simulink model "simpleMicrogrid_PhasorEMT"  (R2017b)
settings: Solver=ode23tb  StartTime=0.0  StopTime=60  RelTol=1e-3
InitFcn:
  | Ts = 1e-4;
  | Rs = 4;
  | Ls = 0;
  | kv = 1;
undefined symbols (not defined in the file): DiscIntNeverNeededParam, Tlim
libraries: powerlib x65, powerlib_meascontrol x7, simulink x6, sps_avr x1, spsDieselMotorModel x1
(part 1 of 2)
settings Model: SimulationMode=accelerator  Creator=jlesage  LastModifiedBy=jlesage
settings DebuggingCC: UnconnectedInputMsg=none  UnconnectedOutputMsg=none  UnconnectedLineMsg=none

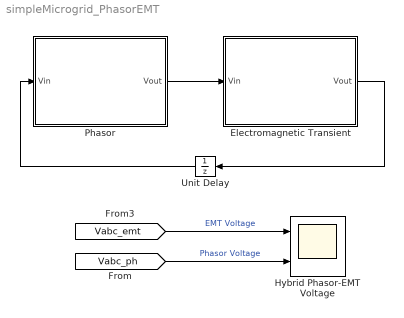
== system simpleMicrogrid_PhasorEMT ==
  Electromagnetic Transient : Subsystem
  Hybrid Phasor-EMT Voltage : Scope  NumInputPorts=2
  Phasor : Subsystem
  Unit Delay : UnitDelay  SampleTime=Ts
  wires:
  Phasor/1(Vout) -> Electromagnetic Transient/1(Vin)
  Electromagnetic Transient/1(Vout) -> Unit Delay/1
  Unit Delay/1 -> Phasor/1(Vin)
  [Vabc_emt] -> Hybrid Phasor-EMT Voltage/1  "EMT Voltage"
  [Vabc_ph] -> Hybrid Phasor-EMT Voltage/2  "Phasor Voltage"

== system simpleMicrogrid_PhasorEMT/Electromagnetic Transient ==
  Vin : Inport  SampleTime=Ts
  Energy Storage : Subsystem  mask(Grid-connected Energy Storage (PQ Model)){Vn=5000, Fn=60, PnomkW=500, kWh_Rated=100, Efficiency=96, LimitVec=[90 10], RechargeSOC=11, Precharge=50, autoRecharge=off, Initial_kWh_pc=80, PQvec=[500e3 0]}
      mask prompts: Vn "Nominal L-L Voltage [Vrms]"; Fn "Nominal Frequency [Hz]"; PnomkW "Rated Power [kW]"; kWh_Rated "Rated Capacity [kWh]"; Efficiency "Overall System Efficiency [%]"; LimitVec "Upper/Lower Charge Limits [%]"; RechargeSOC "SOC to Recharge [%]"; Precharge "Recharge Rate [% of Rated Power]"; autoRecharge "Enable Auto-Recharge"; Initial_kWh_pc "Initial State-of-Charge [0-100%]"; PQvec "Initial Active/Reactive Cmds"
      mask help:
      | The energy storage block models a generic grid-connected energy storage system (ESS), most commonly a battery system. This is a system-level model that does not contain any power electronics, but is useful for load flow, phasor, and hybrid phasor-EMT simulations. The inputs to this block are the commanded active and reactive power of the ESS. The ESS is assumed to have four quadrent operation.
      |
      | For more detailed ESS models, consider the battery block in the Drives library. Consider using this PQ Model to perform load flow studies and switch to a more detailed model when full EMT studies or more advanced controls are required.
      |
      | Note: The initial active/reactive power commands must be specified for use for Load Flow analysis.
      mask init:
      | % Calculate Initial Conditions
      | Pnom = PnomkW*1e3;
      | P0 = -PQvec(1);  Q0 = -PQvec(2);
      | if abs(P0) > Pnom
      |     P0 = sign(P0)*Pnom;
      | end
      | 
      | % Calculate Q0 given Reactive Power Capability Curve
      | Qlim = sqrt(Pnom^2 - P0^2);
      | if Qlim > abs(Q0)
      |     Q0 = sign(Q0)*Qlim;
      | end
      | 
      | UpChrgLim = LimitVec(1);
      | LowChrgLim = LimitVec(2);
      | if Initial_kWh_pc > UpChrgLim && P0 < 0
      |     P0 = 0; Q0 = 0;
      | elseif Initial_kWh_pc < LowChrgLim && P0 > 0
      |     P0 = 0; Q0 = 0;
      | end
      mask DialogControl Container7 Prompt: Grid Connection Properties
      mask DialogControl Container11 Prompt: Charge/Discharge Controls
      mask DialogControl Container12 Prompt: Initial Conditions
  Pref : Constant  Value=100e3
  Qref : Constant  Value=0
  SPS-Simulink Interface : Subsystem  Variant=on  OverrideUsingVariant=EMT  mask(SPS-to-Simulink Voltage Interface){replayType=EMT Replay, Freq=60, kv=kv, Rs=Rs, Ls=Ls, Ts=Ts}
      mask prompts: replayType "Replay Type"; Freq "Nominal Frequency [Hz]"; kv "Voltage Stability Factor, kv"; Rs "Series Resistance, Rs"; Ls "Series Inductance, Ls"; Ts "Sample Time, Ts"
      mask help:
      | This block uses voltage transfer theory to segment a Simscape Power Systems network into subsystems. These subsystems can execute a multiple rates, use Phasor/EMT simulation methods, and run on multiple cores for real-time simulation.
      |
      | Make sure to select the same simulation technique as the powergui setting in the same subsystem.
      mask init:
      | simulationStatus =  get_param(bdroot,'SimulationStatus');
      | 
      | % The active variant can only be modified at edit-time or very early during
      | % the simulink compile stage. 
      | if any(strcmp(simulationStatus, {'stopped'}))
      |     vssBlk = gcb;
      |     freqBlk = [vssBlk '/EMT/Frequency Generator'];
      | 
      |     if strcmp(replayType,'EMT Replay')
      |         set_param(vssBlk, 'OverrideUsingVariant', 'EMT');
      |     else
      |         set_param(vssBlk, 'OverrideUsingVariant', 'Phasor');
      |     end
      |     
      |     if Ts ~= 0
      |         set_param(freqBlk,'OverrideUsingVariant', 'Discrete');
      |     else
      |         set_param(freqBlk, 'OverrideUsingVariant', 'Continuous');
      |     end
      | end
      mask TypeOptions replayType: EMT Replay | Phasor Replay
  Scope : Subsystem
  Three-Phase V-I Measurement : powerlib/Measurements/Three-Phase V-I Measurement  VoltageMeasurement=phase-to-ground  SetLabelV=on  LabelV=Vabc_ess  Vpu=off  VpuLL=off  CurrentMeasurement=yes  SetLabelI=on  LabelI=Iabc_ess  Ipu=off  Pbase=100e6  Vbase=500e3  OutputType=Complex  PhasorSimulation=on  PSBequivalent=0
  powergui : powerlib/powergui  Priority=1  SimulationMode=Discrete  SampleTime=Ts  frequency=60  Iterations=50  frequencyindice=60  Pbase=100e6  ErrMax=0.0001  UnitsV=kV  UnitsW=MW  buscounter=3  FunctionMessages=off  echomessages=off  EnableUseOfTLC=off  CurrentSourceSwitches=off  DisableSnubberDevices=off  DisableRonSwitches=off  DisableVfSwitches=off  DisplayEquations=off  SolverType=Tustin/Backward Euler (TBE)  Interpol=off  ExternalGateDelay=off  methode=off  Ts=100  x0status=blocks  SPID=on  SwTol=0  HookPort=off  RestoreLinks=warning  ResistiveCurrentMeasurement=off  Frange=[0:2:500]  Ylog=off  Xlog=on  ShowGrid=off  save=off  variable=ZData  structure=0  ZoomFFT=off  StartTime=0.0  cycles=1  DisplayStyle=1  fundamental=60  FreqAxis=off  MaxFrequency=1000  frequencyindicesteady=1  RmsSteady=1  display=off
  Vout : Outport  SampleTime=Ts
  tag scope: battM=global
  wires:
  SPS-Simulink Interface/1(Vout) -> Vout/1
  Vin/1 -> SPS-Simulink Interface/1(Vin)
  [Vabc_ess] -> Scope/1(Vrms)
  Energy Storage/1(m) -> [battM]
  Pref/1 -> Energy Storage/1(Pref)
  Qref/1 -> Energy Storage/2(Qref)
  connections:
  Three-Phase V-I Measurement/RConn1 -- Energy Storage/RConn1
  Three-Phase V-I Measurement/RConn2 -- Energy Storage/RConn2
  Three-Phase V-I Measurement/RConn3 -- Energy Storage/RConn3
  Three-Phase V-I Measurement/LConn3 -- SPS-Simulink Interface/RConn3
  Three-Phase V-I Measurement/LConn2 -- SPS-Simulink Interface/RConn2
  Three-Phase V-I Measurement/LConn1 -- SPS-Simulink Interface/RConn1

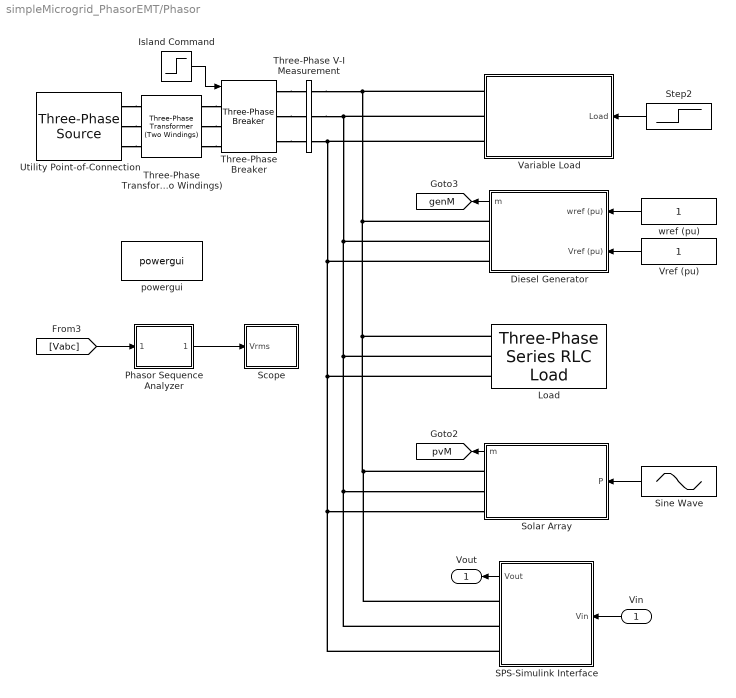
== system simpleMicrogrid_PhasorEMT/Phasor ==
  Vin : Inport
  Diesel Generator : Subsystem  mask(Diesel Generator (Simple)){Pn=1e6, Vn=5000, Fn=60, genType=PQ, PQ0=[0.05 0]}
      mask prompts: Pn "Generator Rated Power [W]"; Vn "Rated Voltage [V]"; Fn "Rated Frequency [Hz]"; genType "Load Flow Type"; PQ0 "Initial Power, [P0 Q0] [pu]"
      mask help:
      | The Diesel Generator block contains a synchronous generator, diesel governor and excitation system to represent the dynamics of a Genset. To inspect the model, look under the block mask (Ctrl + u).
      |
      | The inputs to the basic Diesel generator block are the desired speed reference (in pu) and the desired voltage reference (in pu). The output measurements are contained in a Simulink bus, which can be selected by using the Bus Selector block.
      |
      | Note: The initial generator power must be specified for use for Load Flow analysis.
      mask init:
      | % Extract Initial Active/Reactive Power
      | P0 = PQ0(1);
      | Q0 = PQ0(2);
      | 
      | % Select Load Flow Type
      | genBlock = [gcb '/Synchronous Machine'];
      | currentVals = get_param(genBlock,'MaskValues');
      | currentVals{31} = genType;
      | set_param(genBlock,'MaskValues',currentVals);
      | 
      | % Disable Option if Swing Generator Selected
      | currentEnables = get_param(gcb,'MaskEnables');
      | if strcmp(genType,'swing')
      |     currentEnables{5} = 'off';
      | else
      |     currentEnables{5} = 'on';
      | end
      | set_param(gcb,'MaskEnables',currentEnables);
      settings: AttributesFormatString=Rated Power: %<Pn> W
      mask TypeOptions genType: swing | PQ | PV
      mask Display: %image(imread('diesel.jpg'))
  Island Command : Step  Time=15  Before=1  After=0  SampleTime=0
  Load : powerlib/Elements/Three-Phase Series RLC Load  LConnTagsString=A|B|C  Configuration=Y (grounded)  NominalVoltage=5000  Vabc=[1e3 1e3 1e3]  Vabcp=[1e3 1e3 1e3]  NominalFrequency=60  UnbalancedPower=off  ActivePower=500e3  InductivePower=0  CapacitivePower=0  Pabc=[10e3 9e3 11e3]  QLabc=[100 90 110]  QCabc=[100 90 110]  Pabcp=[10e3 9e3 11e3]  QLabcp=[100 90 110]  QCabcp=[100 90 110]  Measurements=None  LoadType=constant Z
      settings: AttributesFormatString=P = %<ActivePower> W
  Phasor Sequence Analyzer : Subsystem
  SPS-Simulink Interface : Subsystem  Variant=on  OverrideUsingVariant=Phasor  mask(SPS-to-Simulink Voltage Interface){replayType=Phasor Replay, Freq=60, kv=kv, Rs=Rs, Ls=Ls, Ts=Ts}
      mask prompts: replayType "Replay Type"; Freq "Nominal Frequency [Hz]"; kv "Voltage Stability Factor, kv"; Rs "Series Resistance, Rs"; Ls "Series Inductance, Ls"; Ts "Sample Time, Ts"
      mask help:
      | This block uses voltage transfer theory to segment a Simscape Power Systems network into subsystems. These subsystems can execute a multiple rates, use Phasor/EMT simulation methods, and run on multiple cores for real-time simulation.
      |
      | Make sure to select the same simulation technique as the powergui setting in the same subsystem.
      mask init: same as simpleMicrogrid_PhasorEMT/Electromagnetic Transient/SPS-Simulink Interface
      mask TypeOptions replayType: EMT Replay | Phasor Replay
  Scope : Subsystem
  Sine Wave : Sin  Amplitude=200e3  Bias=250e3  Frequency=0.05  SampleTime=0
  Solar Array : Subsystem  mask(Grid-Connected PV Array (PQ Model)){Vn=5000, Fn=60, P0=500e3}
      mask prompts: Vn "Nominal L-L Voltage [Vrms]"; Fn "Nominal Frequency [Hz]"; P0 "Initial Power [W]"
      mask help:
      | This block models a grid-connected solar array using the Three-Phase Dynamic Load block. This is a system-level model that does not contain any power electronics, but is useful for load flow, phasor, and hybrid phasor-EMT simulations. The input to this block is the power output of the grid connected PV array, not irradiance.
      |
      | For more detailed PV models, consider the PV Array block in the Renewables library. Consider using this PQ Model to perform load flow studies and switch to a more detailed model when full EMT studies are required.
      |
      | Note: The array power must be specified for use for Load Flow analysis.
      mask init:
      | % P0 = Irr0*TotalArea*Efficiency/100;
      | P0 = -P0;
      mask Display:
      | image(imread('PV_Farm.jpg'))
      | color('white')
      | port_label('input',1,'P')
      | port_label('output',1,'m')
      | port_label('Rconn',1,'A')
      | port_label('Rconn',2,'B')
      | port_label('Rconn',3,'C')
  Step2 : Step  Time=35  Before=200e3  After=500e3  SampleTime=0
  Three-Phase Transformer (Two Windings) : powerlib/Elements/Three-Phase Transformer (Two Windings)  Winding1Connection=Yg  Winding2Connection=Yg  CoreType=Three single-phase transformers  SetSaturation=off  Hysteresis=off  DataFile='hysteresis'  SetInitialFlux=off  Measurements=None  UNITS=pu  NominalPower=[ 250e6 , 60 ]  Winding1=[ 13.8e3 , 0.002 , 0.08 ]  Winding2=[ 5000 , 0.002 , 0.08 ]  Rm=500  Lm=500  L0=0.5  Saturation=[ 0,0 ; 0.0024,1.2 ; 1.0,1.52 ]  InitialFluxes=[ 0.8 , -0.8 , 0.7 ]  MoreParameters=off  BreakLoop=off  DataType=off  TransfoNumber=1
  Three-Phase V-I Measurement : powerlib/Measurements/Three-Phase V-I Measurement  VoltageMeasurement=phase-to-ground  SetLabelV=on  LabelV=Vabc  Vpu=off  VpuLL=off  CurrentMeasurement=yes  SetLabelI=on  LabelI=Iabc  Ipu=off  Pbase=100e6  Vbase=500e3  OutputType=Complex  PhasorSimulation=on  PSBequivalent=0
  Three-Phase Breaker : powerlib/Elements/Three-Phase Breaker  InitialState=closed  SwitchA=on  SwitchB=on  SwitchC=on  SwitchTimes="[1/60  5/60]"  External=on  BreakerResistance=0.01  SnubberResistance=1e6  SnubberCapacitance=inf  Measurements=None
  Utility Point-of-Connection : powerlib/Electrical Sources/Three-Phase Source  InternalConnection=Yg  VoltagePhases=off  Voltage=(13800)*1.00243  PhaseAngle=0.071468  Voltage_phases=[25e3 25e3 25e3]/sqrt(3)  PhaseAngles_phases=[0 -120 +120]  Frequency=60  NonIdealSource=on  SpecifyImpedance=on  Resistance=0.8929  Inductance=16.58e-3  ShortCircuitLevel=250e6  BaseVoltage=13.8e3  XRratio=7  BusType=swing  Pref=10e3  Qref=0  Prefabc=[10e3, 10e3, 10e3]  Qrefabc=[0, 0, 0]  Qmin=-inf  Qmax=inf
  Variable Load : Subsystem  mask(Variable Load (PQ Model)){Vn=5000, Fn=60, PF=1, Load0=200e3}
      mask prompts: Vn "Nominal L-L Voltage [Vrms]"; Fn "Nominal Frequency [Hz]"; PF "Power Factor [0 to 1]"; Load0 "Initial Load [W]"
      mask help:
      | The Variable Load block is a lumped approximation for a distribution feeder. For non-unity power factor loads, the input (active power) is scaled accordingly to generate a desired load.
      |
      | Note: The initial input load must be specified for use for Load Flow analysis.
      mask init:
      | P0 = Load0;
      | Q0 = Load0*sqrt(1/PF-1);
      mask Display:
      | image(imread('Residential.jpg'))
      | color('white')
      | port_label('input',1,'Load')
      | port_label('Rconn',1,'A')
      | port_label('Rconn',2,'B')
      | port_label('Rconn',3,'C')
  Vref (pu) : Constant
  powergui : powerlib/powergui  Priority=1  SimulationMode=Phasor  SampleTime=1e-4  frequency=60  Iterations=50  frequencyindice=60  Pbase=100e6  ErrMax=0.0001  UnitsV=kV  UnitsW=MW  buscounter=3  FunctionMessages=off  echomessages=off  EnableUseOfTLC=off  CurrentSourceSwitches=off  DisableSnubberDevices=off  DisableRonSwitches=off  DisableVfSwitches=off  DisplayEquations=off  SolverType=Tustin/Backward Euler (TBE)  Interpol=off  ExternalGateDelay=off  methode=off  Ts=100  x0status=blocks  SPID=on  SwTol=0  HookPort=off  RestoreLinks=warning  ResistiveCurrentMeasurement=off  Frange=[0:2:500]  Ylog=off  Xlog=on  ShowGrid=off  save=off  variable=ZData  structure=0  ZoomFFT=off  StartTime=0.0  cycles=1  DisplayStyle=1  fundamental=60  FreqAxis=off  MaxFrequency=1000  frequencyindicesteady=1  RmsSteady=1  display=off
  wref (pu) : Constant
  Vout : Outport
  tag scope: genM=global, pvM=global
  wires:
  Vref (pu)/1 -> Diesel Generator/2(Vref (pu))
  wref (pu)/1 -> Diesel Generator/1(wref (pu))
  Island Command/1 -> Three-Phase Breaker/1
  Sine Wave/1 -> Solar Array/1(P)
  Phasor Sequence Analyzer/1(Vrms) -> Scope/1(Vrms)
  [Vabc] -> Phasor Sequence Analyzer/1(Vabc)
  Diesel Generator/1(m) -> [genM]
  Step2/1 -> Variable Load/1(Load)
  Solar Array/1(m) -> [pvM]
  Vin/1 -> SPS-Simulink Interface/1(Vin)
  SPS-Simulink Interface/1(Vout) -> Vout/1
  connections:
  Utility Point-of-Connection/RConn1 -- Three-Phase Transformer (Two Windings)/LConn1
  Utility Point-of-Connection/RConn3 -- Three-Phase Transformer (Two Windings)/LConn3
  Three-Phase Transformer (Two Windings)/RConn1 -- Three-Phase Breaker/LConn1
  Three-Phase Transformer (Two Windings)/RConn2 -- Three-Phase Breaker/LConn2
  Utility Point-of-Connection/RConn2 -- Three-Phase Transformer (Two Windings)/LConn2
  Three-Phase Transformer (Two Windings)/RConn3 -- Three-Phase Breaker/LConn3
  Variable Load/RConn1 -- Three-Phase V-I Measurement/RConn1 -- Load/LConn1 -- SPS-Simulink Interface/RConn1 -- Solar Array/RConn1 -- Diesel Generator/RConn1
  SPS-Simulink Interface/RConn2 -- Solar Array/RConn2 -- Load/LConn2 -- Three-Phase V-I Measurement/RConn2 -- Variable Load/RConn2 -- Diesel Generator/RConn2
  SPS-Simulink Interface/RConn3 -- Solar Array/RConn3 -- Load/LConn3 -- Three-Phase V-I Measurement/RConn3 -- Variable Load/RConn3 -- Diesel Generator/RConn3
  Three-Phase Breaker/RConn1 -- Three-Phase V-I Measurement/LConn1
  Three-Phase Breaker/RConn3 -- Three-Phase V-I Measurement/LConn3
  Three-Phase Breaker/RConn2 -- Three-Phase V-I Measurement/LConn2

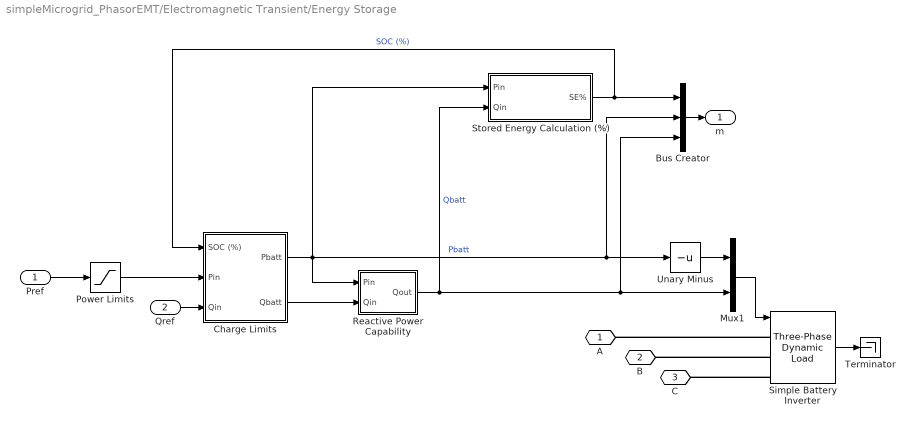
== system simpleMicrogrid_PhasorEMT/Electromagnetic Transient/Energy Storage ==
  Pref : Inport  SampleTime=Ts
  Qref : Inport  Port=2  SampleTime=Ts
  Bus Creator : BusCreator  Inputs=3
  Charge Limits : Subsystem
  Mux1 : Mux  Inputs=2
  Power Limits : Saturate  UpperLimit=Pnom  LowerLimit=-Pnom
  Reactive Power Capability : Subsystem
  Simple Battery Inverter : powerlib/Elements/Three-Phase Dynamic Load  NominalVoltage=[Vn Fn]  ActiveReactivePowers=[-500000 -3.38813e-13]  PositiveSequence=[0.999844 -0.0038635]  ExternalControl=on  NpNq=[1.3 2]  TimeConstants="[0  0  0  0]"  MinimumVoltage=0.7  Tfilter=1e-2  LoadFlowParameters=[4,0,0,0,0]
      settings: SourceProductName=Simscape Power Systems  SourceProductBaseCode=PS
  Stored Energy Calculation (%) : Subsystem
  Terminator : Terminator
  Unary Minus : UnaryMinus
  A : PMIOPort  Port=1  Side=Right
  B : PMIOPort  Port=2  Side=Right
  C : PMIOPort  Port=3  Side=Right
  m : Outport
  wires:
  Charge Limits/2(Qbatt) -> Reactive Power Capability/2(Qin)
  Qref/1 -> Charge Limits/3(Qin)
  Power Limits/1 -> Charge Limits/2(Pin)
  Charge Limits/1(Pbatt) -> Reactive Power Capability/1(Pin), Unary Minus/1, Bus Creator/2, Stored Energy Calculation (%)/1(Pin)  "Pbatt"
  Stored Energy Calculation (%)/1(SE%) -> Bus Creator/1, Charge Limits/1(SOC (%))  "SOC (%)"
  Bus Creator/1 -> m/1
  Pref/1 -> Power Limits/1
  Reactive Power Capability/1(Qout) -> Mux1/2, Bus Creator/3, Stored Energy Calculation (%)/2(Qin)  "Qbatt"
  Simple Battery Inverter/1 -> Terminator/1
  Mux1/1 -> Simple Battery Inverter/1
  Unary Minus/1 -> Mux1/1
  connections:
  Simple Battery Inverter/LConn1 -- A/RConn1
  Simple Battery Inverter/LConn3 -- C/RConn1
  Simple Battery Inverter/LConn2 -- B/RConn1

== system simpleMicrogrid_PhasorEMT/Electromagnetic Transient/SPS-Simulink Interface ==
  Vin : Inport
  EMT : Subsystem  VariantControl=EMT
  Phasor : Subsystem  VariantControl=Phasor
  A : PMIOPort  Port=1  Side=Right
  B : PMIOPort  Port=2  Side=Right
  C : PMIOPort  Port=3  Side=Right
  Vout : Outport

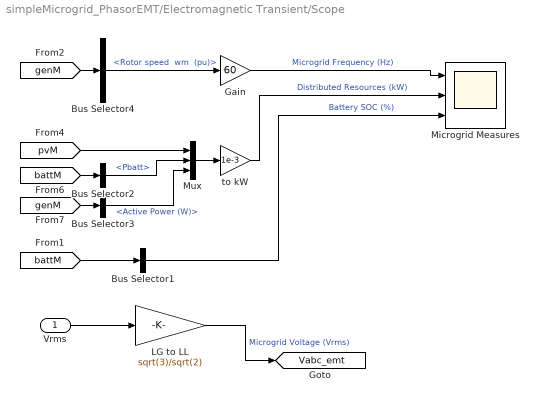
== system simpleMicrogrid_PhasorEMT/Electromagnetic Transient/Scope ==
  Vrms : Inport
  Bus Selector1 : BusSelector  OutputSignals=SOC (%)  OutputAsBus=on
  Bus Selector2 : BusSelector  OutputSignals=Pbatt
  Bus Selector3 : BusSelector  OutputSignals=Active Power (W)
  Bus Selector4 : BusSelector  OutputSignals="Rotor speed  wm  (pu)"
  Gain : Gain  Gain=60
  LG to LL : Gain  Gain=sqrt(3)/sqrt(2)
  Microgrid Measures : Scope  NumInputPorts=3
  Mux : Mux  Inputs=3
  to kW : Gain  Gain=1e-3
  tag scope: Vabc_emt=global
  wires:
  Vrms/1 -> LG to LL/1
  LG to LL/1 -> [Vabc_emt]  "Microgrid Voltage (Vrms)"
  Mux/1 -> to kW/1
  [pvM] -> Mux/1
  Bus Selector2/1 -> Mux/2  "<Pbatt>"
  [battM] -> Bus Selector2/1
  [genM] -> Bus Selector3/1
  [battM] -> Bus Selector1/1
  Bus Selector1/1 -> Microgrid Measures/3  "Battery SOC (%)"
  Gain/1 -> Microgrid Measures/1  "Microgrid Frequency (Hz)"
  [genM] -> Bus Selector4/1
  Bus Selector4/1 -> Gain/1  "<Rotor speed  wm  (pu)>"
  to kW/1 -> Microgrid Measures/2  "Distributed Resources (kW)"
  Bus Selector3/1 -> Mux/3  "<Active Power (W)>"

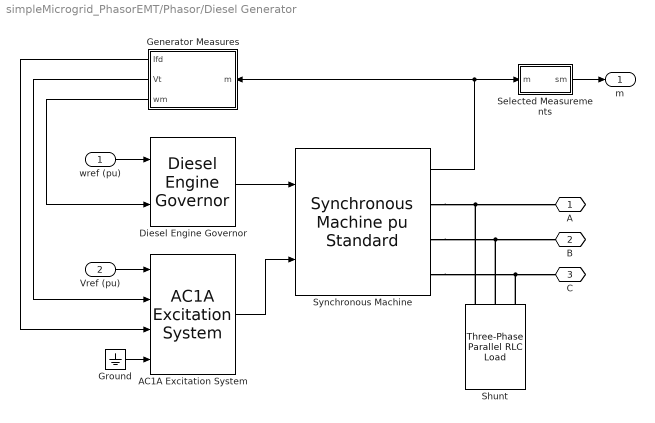
== system simpleMicrogrid_PhasorEMT/Phasor/Diesel Generator ==
  wref (pu) : Inport
  Vref (pu) : Inport  Port=2
  AC1A Excitation System : sps_avr/AC1A Excitation System  Tr=20e-3  KaTa=[400 0.02]  VAminmax=[-14.5 14.5]  VRminmax=[-5.43 6.03]  KfTf=[0.03 1.0]  TbTc=[0 0]  KeTe=[1.0 0.80]  Ve12=[4.18 3.14]  SeVe12=[0.10 0.03]  Kd=0.38  Kc=0.20  v0=[0.99984 1.0013]  TsBlock=0
      settings: SourceProductName=Simscape Power Systems  SourceProductBaseCode=PS
  Diesel Engine Governor : spsDieselMotorModel/Diesel Engine Governor  K=29  Tr=[0.01 0.02 0.2]  Ta=[0.25 0.009 0.0384]  Tlim=[0 1.1]  Td=0.024  Pm0=0.050008
  Generator Measures : Subsystem
  Ground : Ground
  Selected Measurements : Subsystem
  Shunt : powerlib/Elements/Three-Phase Parallel RLC Load  LConnTagsString=A|B|C  Configuration=Y (grounded)  NominalVoltage=Vn  Vabc=[1e3 1e3 1e3]  Vabcp=[1e3 1e3 1e3]  NominalFrequency=Fn  UnbalancedPower=off  ActivePower=Pn*0.05  InductivePower=0  CapacitivePower=0  Pabc=[10e3 9e3 11e3]  QLabc=[100 90 110]  QCabc=[100 90 110]  Pabcp=[10e3 9e3 11e3]  QLabcp=[100 90 110]  QCabcp=[100 90 110]  Measurements=None  LoadType=constant Z
  Synchronous Machine : powerlib/Machines/Synchronous Machine pu Standard  PresetModel=No  MechanicalLoad=Mechanical power Pm  ShowDetailedParameters=on  RotorType=Salient-pole  Units=per unit standard parameters  MeasurementBus=off  NominalParameters=[ Pn Vn Fn]  Reactances1=[ 1.81, 0.3, 0.23, 1.76, 0.65, 0.25, 0.15 ]  Reactances2="[ 1.305, 0.296, 0.252, 0.474,  0.243,  0.18 ]"  dAxisTimeConstants=Open-circuit  qAxisTimeConstants=Short-circuit  TimeConstants1="[ 4.4849  0.0681  0.1  ]"  TimeConstants2=[ 8.0, 0.03, 1.0, 0.07 ]  TimeConstants3="[  4.49  0.0681  0.0513  ]"  TimeConstants4=[ 8.0, 0.03, 0.3371, 0.0295 ]  TimeConstants5=[ 1.01, 0.053, 0.1 ]  TimeConstants6=[ 1.3201, 0.023, 1.0, 0.07 ]  TimeConstants7=[0.012 0.003 0.003]  TimeConstants8=[ 1.3201, 0.0231, 0.3371, 0.0295 ]  StatorResistance=0.003  Mechanical=[3.7 0 1 ]  PolePairs=20  InitialConditions=[0 -88.646 0.0500078 0.0500078 0.0500078 -0.0038635 -120.004 119.996 1.00126]  SetSaturation=off  Saturation=[0.6404,0.7127,0.8441,0.9214,0.9956,1.082,1.19,1.316,1.457;0.7,0.7698,0.8872,0.9466,0.9969,1.046,1.1,1.151,1.201]  LoadFlowParameters=[1,0,0,0,0]  TsPowergui=0  TsBlock=-1  IterativeModel=Trapezoidal non iterative  IterativeDiscreteModel=Trapezoidal non iterative  BusType=PQ  Pref=Pn*P0  Qref=0  Qmin=-inf  Qmax=inf  PLF=0  QLF=0
      settings: SourceProductName=Simscape Power Systems
  A : PMIOPort  Port=1  Side=Right
  B : PMIOPort  Port=2  Side=Right
  C : PMIOPort  Port=3  Side=Right
  m : Outport
  wires:
  wref (pu)/1 -> Diesel Engine Governor/1
  Diesel Engine Governor/1 -> Synchronous Machine/1
  AC1A Excitation System/1 -> Synchronous Machine/2
  Vref (pu)/1 -> AC1A Excitation System/1
  Synchronous Machine/1 -> Generator Measures/1(m), Selected Measurements/1(m)
  Ground/1 -> AC1A Excitation System/4
  Generator Measures/3(wm) -> Diesel Engine Governor/2
  Generator Measures/2(Vt) -> AC1A Excitation System/2
  Generator Measures/1(Ifd) -> AC1A Excitation System/3
  Selected Measurements/1(sm) -> m/1
  connections:
  Shunt/LConn1 -- Synchronous Machine/RConn1 -- A/RConn1
  Synchronous Machine/RConn3 -- Shunt/LConn3 -- C/RConn1
  Synchronous Machine/RConn2 -- Shunt/LConn2 -- B/RConn1

== system simpleMicrogrid_PhasorEMT/Phasor/Phasor Sequence Analyzer ==
  Vabc : Inport
  Sequence Analyzer (Phasor) : powerlib_meascontrol/Measurements/Sequence Analyzer (Phasor)  seq=Positive
      settings: SourceProductName=Simscape Power Systems  SourceProductBaseCode=PS
  Terminator : Terminator
  Vrms : Outport
  wires:
  Sequence Analyzer (Phasor)/1 -> Vrms/1
  Vabc/1 -> Sequence Analyzer (Phasor)/1
  Sequence Analyzer (Phasor)/2 -> Terminator/1

== system simpleMicrogrid_PhasorEMT/Phasor/SPS-Simulink Interface ==
  Vin : Inport
  EMT : Subsystem  VariantControl=EMT
  Phasor : Subsystem  VariantControl=Phasor
  A : PMIOPort  Port=1  Side=Right
  B : PMIOPort  Port=2  Side=Right
  C : PMIOPort  Port=3  Side=Right
  Vout : Outport

== system simpleMicrogrid_PhasorEMT/Phasor/Scope ==
  Vrms : Inport
  LG to LL : Gain  Gain=sqrt(3)/sqrt(2)
  tag scope: Vabc_ph=global
  wires:
  LG to LL/1 -> [Vabc_ph]  "Microgrid Voltage (Vrms)"
  Vrms/1 -> LG to LL/1

== system simpleMicrogrid_PhasorEMT/Phasor/Solar Array ==
  P : Inport
  Bus Selector : BusSelector  OutputSignals=Active power P (W)
  Constant11 : Constant  Value=0
  Mux1 : Mux  Inputs=2
  Simple Solar Inverter : powerlib/Elements/Three-Phase Dynamic Load  NominalVoltage=[Vn Fn]  ActiveReactivePowers=[-250000 -3.38813e-13]  PositiveSequence=[0.999844 -0.0038635]  ExternalControl=on  NpNq=[1.3 2]  TimeConstants="[0  0  0  0]"  MinimumVoltage=0.7  Tfilter=1e-2  LoadFlowParameters=[4,0,0,0,0]
      settings: SourceProductName=Simscape Power Systems  SourceProductBaseCode=PS
  Unary Minus : UnaryMinus
  Unary Minus1 : UnaryMinus
  A : PMIOPort  Port=1  Side=Right
  B : PMIOPort  Port=2  Side=Right
  C : PMIOPort  Port=3  Side=Right
  m : Outport
  wires:
  P/1 -> Unary Minus/1
  Unary Minus/1 -> Mux1/1
  Mux1/1 -> Simple Solar Inverter/1
  Constant11/1 -> Mux1/2
  Simple Solar Inverter/1 -> Bus Selector/1
  Bus Selector/1 -> Unary Minus1/1  "<Active power P (W)>"
  Unary Minus1/1 -> m/1
  connections:
  Simple Solar Inverter/LConn2 -- B/RConn1
  Simple Solar Inverter/LConn3 -- C/RConn1
  Simple Solar Inverter/LConn1 -- A/RConn1

== system simpleMicrogrid_PhasorEMT/Phasor/Variable Load ==
  Load : Inport
  Dynamic Load Control : Subsystem
  Simple Three-Phase Load : powerlib/Elements/Three-Phase Dynamic Load  NominalVoltage=[Vn Fn]  ActiveReactivePowers=[200000 45883.1]  PositiveSequence=[0.999844 -0.0038635]  ExternalControl=on  NpNq=[1.3 2]  TimeConstants="[0  0  0  0]"  MinimumVoltage=0.7  Tfilter=1e-2  LoadFlowParameters=[4,0,0,0,0]
      settings: SourceProductName=Simscape Power Systems  SourceProductBaseCode=PS
  Terminator : Terminator
  A : PMIOPort  Port=1  Side=Right
  B : PMIOPort  Port=2  Side=Right
  C : PMIOPort  Port=3  Side=Right
  wires:
  Simple Three-Phase Load/1 -> Terminator/1
  Load/1 -> Dynamic Load Control/1(P0)
  Dynamic Load Control/1(PQ) -> Simple Three-Phase Load/1
  connections:
  Simple Three-Phase Load/LConn1 -- A/RConn1
  Simple Three-Phase Load/LConn3 -- C/RConn1
  Simple Three-Phase Load/LConn2 -- B/RConn1

== system simpleMicrogrid_PhasorEMT/Electromagnetic Transient/Energy Storage/Charge Limits ==
  SOC (%) : Inport
  Pin : Inport  Port=2
  Qin : Inport  Port=3
  Overcharge Check : Subsystem
  Undercharge Check : Subsystem
  Pbatt : Outport
  Qbatt : Outport  Port=2
  wires:
  SOC (%)/1 -> Overcharge Check/1(SOC (%)), Undercharge Check/1(SOC (%))
  Undercharge Check/2(Qout) -> Qbatt/1
  Pin/1 -> Overcharge Check/2(Pin)
  Overcharge Check/1(Pout) -> Undercharge Check/2(Pin)
  Qin/1 -> Overcharge Check/3(Qin)
  Undercharge Check/1(Pout) -> Pbatt/1  "Pbatt"
  Overcharge Check/2(Qout) -> Undercharge Check/3(Qin)

== system simpleMicrogrid_PhasorEMT/Electromagnetic Transient/Energy Storage/Reactive Power Capability ==
  Pin : Inport
  Qin : Inport  Port=2
  Constant : Constant  Value=Pnom
  Math Function : Math  Operator=square  SaturateOnIntegerOverflow=on
  Math Function1 : Math  Operator=square  SaturateOnIntegerOverflow=on
  Saturation Dynamic : simulink/Discontinuities/Saturation Dynamic  OutMin=[]  OutMax=[]  OutDataTypeStr=Inherit: Same as second input  OutDataType=fixdt(1, 16)  OutScaling=2^-10  DoSatur=off
  Sqrt : Sqrt  SaturateOnIntegerOverflow=on
  Sum : Sum  Inputs=-+|
  Unary Minus : UnaryMinus
  Qout : Outport
  wires:
  Sqrt/1 -> Saturation Dynamic/1, Unary Minus/1
  Math Function1/1 -> Sum/1
  Math Function/1 -> Sum/2
  Constant/1 -> Math Function/1
  Sum/1 -> Sqrt/1
  Unary Minus/1 -> Saturation Dynamic/3
  Saturation Dynamic/1 -> Qout/1
  Pin/1 -> Math Function1/1
  Qin/1 -> Saturation Dynamic/2

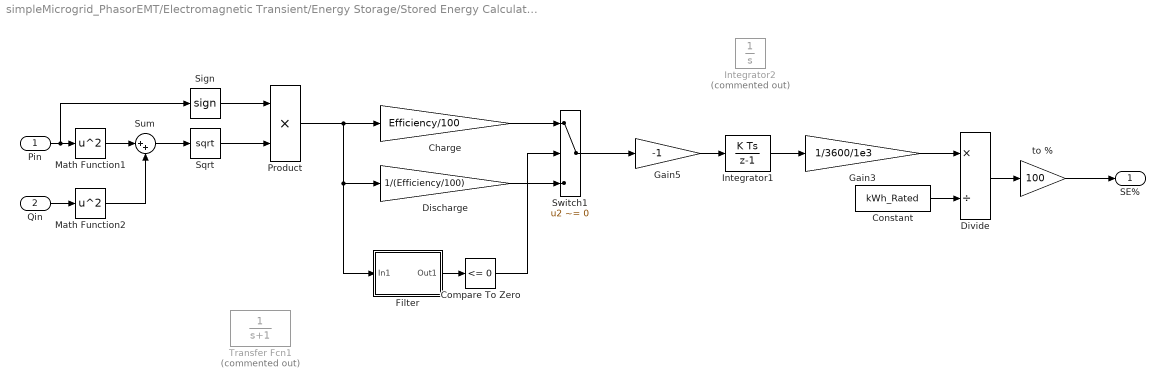
== system simpleMicrogrid_PhasorEMT/Electromagnetic Transient/Energy Storage/Stored Energy Calculation (%) ==
  Pin : Inport
  Qin : Inport  Port=2
  Charge : Gain  Gain=Efficiency/100
  Compare To Zero : simulink/Logic and Bit Operations/Compare To Zero  relop=<=  OutDataTypeStr=boolean
  Constant : Constant  Value=kWh_Rated
  Discharge : Gain  Gain=1/(Efficiency/100)
  Divide : Product  Inputs=*/
  Filter : Subsystem  mask{Tf=1}
      mask prompts: Tf "Time Constant, Tf"
      mask Display: fprintf('1\n------------\n(1 + s Tf)');
  Gain3 : Gain  Gain=1/3600/1e3
  Gain5 : Gain  Gain=-1
  Integrator1 : DiscreteIntegrator  InitialCondition=(Initial_kWh_pc/100)*kWh_Rated*3600*1e3  SampleTime=Ts  UpperSaturationLimit=Tlim(2)  LowerSaturationLimit=Tlim(1)  ICPrevOutput=DiscIntNeverNeededParam  ICPrevScaledInput=DiscIntNeverNeededParam
  Integrator2 : Integrator  Commented=on  InitialCondition=(Initial_kWh_pc/100)*kWh_Rated*3600*1e3
  Math Function1 : Math  Operator=square  SaturateOnIntegerOverflow=on
  Math Function2 : Math  Operator=square  SaturateOnIntegerOverflow=on
  Product : Product
  Sign : Signum
  Sqrt : Sqrt  SaturateOnIntegerOverflow=on
  Sum : Sum  Inputs=|++
  Switch1 : Switch  Criteria=u2 ~= 0
  Transfer Fcn1 : TransferFcn  Commented=on  Denominator=[1 1]
  to % : Gain  Gain=100
  SE% : Outport
  wires:
  Sign/1 -> Product/1
  Sqrt/1 -> Product/2
  Sum/1 -> Sqrt/1
  Math Function2/1 -> Sum/2
  Math Function1/1 -> Sum/1
  Qin/1 -> Math Function2/1
  Pin/1 -> Math Function1/1, Sign/1
  Product/1 -> Filter/1(In1), Discharge/1, Charge/1
  Discharge/1 -> Switch1/3
  Gain5/1 -> Integrator1/1
  to %/1 -> SE%/1
  Filter/1(Out1) -> Compare To Zero/1
  Switch1/1 -> Gain5/1
  Gain3/1 -> Divide/1
  Constant/1 -> Divide/2
  Charge/1 -> Switch1/1
  Divide/1 -> to %/1
  Compare To Zero/1 -> Switch1/2
  Integrator1/1 -> Gain3/1

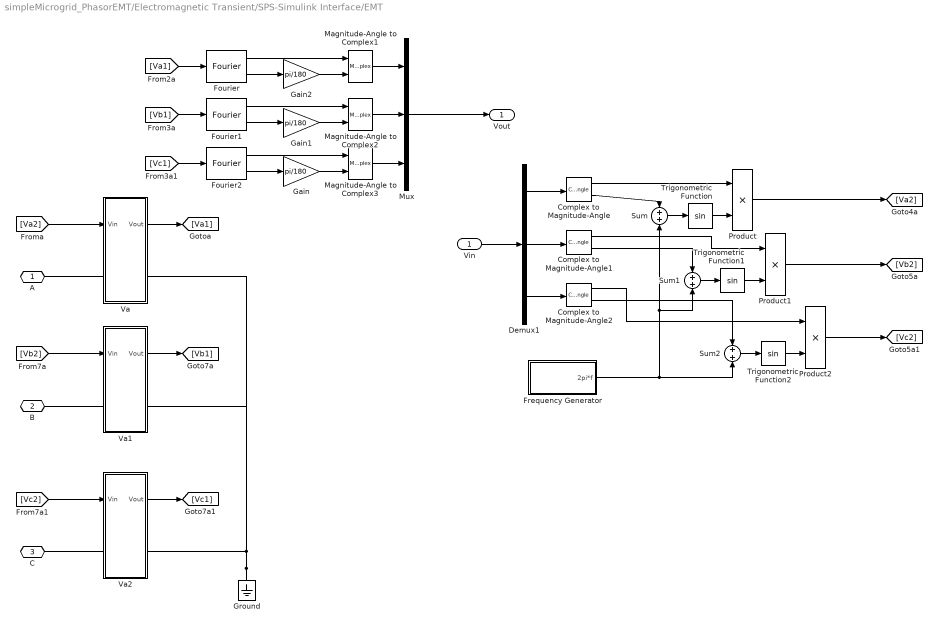
== system simpleMicrogrid_PhasorEMT/Electromagnetic Transient/SPS-Simulink Interface/EMT ==
  Vin : Inport
      settings: SignalType=complex
  Complex to Magnitude-Angle : ComplexToMagnitudeAngle
  Complex to Magnitude-Angle1 : ComplexToMagnitudeAngle
  Complex to Magnitude-Angle2 : ComplexToMagnitudeAngle
  Demux1 : Demux  Outputs=3
  Fourier : powerlib_meascontrol/Measurements/Fourier  Freq=60  n=1  InInit=[1, 0]  Ts=Ts
      settings: SourceProductName=Simscape Power Systems
  Fourier1 : powerlib_meascontrol/Measurements/Fourier  Freq=60  n=1  InInit=[1, 0]  Ts=Ts
      settings: SourceProductName=Simscape Power Systems
  Fourier2 : powerlib_meascontrol/Measurements/Fourier  Freq=60  n=1  InInit=[1, 0]  Ts=Ts
      settings: SourceProductName=Simscape Power Systems
  Frequency Generator : Subsystem  Variant=on  OverrideUsingVariant=Continuous
  Gain : Gain  Gain=pi/180
  Gain1 : Gain  Gain=pi/180
  Gain2 : Gain  Gain=pi/180
  Ground : powerlib/Elements/Ground  LConnTagsString=a
  Magnitude-Angle to Complex1 : MagnitudeAngleToComplex
  Magnitude-Angle to Complex2 : MagnitudeAngleToComplex
  Magnitude-Angle to Complex3 : MagnitudeAngleToComplex
  Mux : Mux  Inputs=3
  Product : Product
  Product1 : Product
  Product2 : Product
  Sum : Sum
  Sum1 : Sum
  Sum2 : Sum
  Trigonometric Function : Trigonometry
  Trigonometric Function1 : Trigonometry
  Trigonometric Function2 : Trigonometry
  Va : Subsystem
  Va1 : Subsystem
  Va2 : Subsystem
  A : PMIOPort  Port=1  Side=Right
  B : PMIOPort  Port=2  Side=Right
  C : PMIOPort  Port=3  Side=Right
  Vout : Outport
      settings: SignalType=complex
  wires:
  Complex to Magnitude-Angle2/2 -> Sum2/1
  Sum2/1 -> Trigonometric Function2/1
  Trigonometric Function2/1 -> Product2/2
  Complex to Magnitude-Angle2/1 -> Product2/1
  Complex to Magnitude-Angle1/1 -> Product1/1
  Trigonometric Function1/1 -> Product1/2
  Sum1/1 -> Trigonometric Function1/1
  Complex to Magnitude-Angle1/2 -> Sum1/1
  Frequency Generator/1(2pi*f) -> Sum/2, Sum1/2, Sum2/2
  Complex to Magnitude-Angle/2 -> Sum/1
  Sum/1 -> Trigonometric Function/1
  Trigonometric Function/1 -> Product/2
  Complex to Magnitude-Angle/1 -> Product/1
  Demux1/3 -> Complex to Magnitude-Angle2/1
  Demux1/2 -> Complex to Magnitude-Angle1/1
  Demux1/1 -> Complex to Magnitude-Angle/1
  Gain2/1 -> Magnitude-Angle to Complex1/2
  Gain1/1 -> Magnitude-Angle to Complex2/2
  Gain/1 -> Magnitude-Angle to Complex3/2
  Magnitude-Angle to Complex2/1 -> Mux/2
  Magnitude-Angle to Complex3/1 -> Mux/3
  Fourier2/2 -> Gain/1
  Fourier2/1 -> Magnitude-Angle to Complex3/1
  Fourier1/2 -> Gain1/1
  Fourier1/1 -> Magnitude-Angle to Complex2/1
  Magnitude-Angle to Complex1/1 -> Mux/1
  Fourier/1 -> Magnitude-Angle to Complex1/1
  Fourier/2 -> Gain2/1
  [Vc1] -> Fourier2/1
  [Vb1] -> Fourier1/1
  [Va1] -> Fourier/1
  Vin/1 -> Demux1/1
  Mux/1 -> Vout/1
  Product/1 -> [Va2]
  Product1/1 -> [Vb2]
  [Va2] -> Va/1(Vin)
  Va/1(Vout) -> [Va1]
  [Vb2] -> Va1/1(Vin)
  Va1/1(Vout) -> [Vb1]
  Va2/1(Vout) -> [Vc1]
  [Vc2] -> Va2/1(Vin)
  Product2/1 -> [Vc2]
  connections:
  Ground/LConn1 -- Va2/RConn1 -- Va1/RConn1 -- Va/RConn1
  Va/LConn1 -- A/RConn1
  Va1/LConn1 -- B/RConn1
  Va2/LConn1 -- C/RConn1

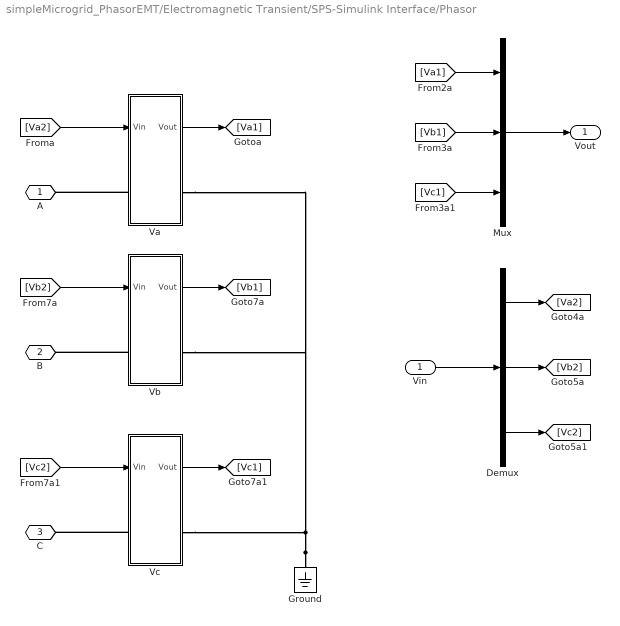
== system simpleMicrogrid_PhasorEMT/Electromagnetic Transient/SPS-Simulink Interface/Phasor ==
  Vin : Inport
  Demux : Demux  Outputs=3
  Ground : powerlib/Elements/Ground  LConnTagsString=a
  Mux : Mux  Inputs=3
  Va : Subsystem
  Vb : Subsystem
  Vc : Subsystem
  A : PMIOPort  Port=1  Side=Right
  B : PMIOPort  Port=2  Side=Right
  C : PMIOPort  Port=3  Side=Right
  Vout : Outport
  wires:
  Vin/1 -> Demux/1
  Mux/1 -> Vout/1
  [Va1] -> Mux/1
  [Vb1] -> Mux/2
  Demux/1 -> [Va2]
  Demux/2 -> [Vb2]
  [Va2] -> Va/1(Vin)
  Va/1(Vout) -> [Va1]
  [Vb2] -> Vb/1(Vin)
  Vb/1(Vout) -> [Vb1]
  Vc/1(Vout) -> [Vc1]
  [Vc2] -> Vc/1(Vin)
  [Vc1] -> Mux/3
  Demux/3 -> [Vc2]
  connections:
  Ground/LConn1 -- Vc/RConn1 -- Vb/RConn1 -- Va/RConn1
  Va/LConn1 -- A/RConn1
  Vb/LConn1 -- B/RConn1
  Vc/LConn1 -- C/RConn1

== system simpleMicrogrid_PhasorEMT/Phasor/Diesel Generator/Generator Measures ==
  m : Inport
  Bus Selector : BusSelector  OutputSignals="dq0 components.Stator voltage  vq (pu),dq0 components.Stator voltage  vd (pu)"  OutputAsBus=on
  Bus Selector1 : BusSelector  OutputSignals="Mechanical.Rotor speed  wm  (pu),dq0 components.Field current  ifd (pu)"
  Fcn1 : Fcn  Expr=sqrt(u(1)^2 + u(2)^2)
  Ifd : Outport
  Vt : Outport  Port=2
  wm : Outport  Port=3
  wires:
  Bus Selector1/1 -> wm/1  "<Rotor speed  wm  (pu)>"
  m/1 -> Bus Selector1/1, Bus Selector/1
  Fcn1/1 -> Vt/1
  Bus Selector/1 -> Fcn1/1
  Bus Selector1/2 -> Ifd/1  "<Field current  ifd (pu)>"

== system simpleMicrogrid_PhasorEMT/Phasor/Diesel Generator/Selected Measurements ==
  m : Inport
  Bus Creator : BusCreator  Inputs=7
  Bus Selector : BusSelector  OutputSignals="Mechanical.Electrical power  Pe (pu),Mechanical.Rotor speed  wm  (pu),Output active power   Peo (pu),Output reactive power  Qeo (pu)"
  to W : Gain  Gain=Pn
  to W1 : Gain  Gain=Pn
  to W2 : Gain  Gain=Pn
  sm : Outport
  wires:
  to W2/1 -> Bus Creator/7  "Reactive Power (W)"
  to W1/1 -> Bus Creator/6  "Active Power (W)"
  Bus Selector/2 -> Bus Creator/3  "<Rotor speed  wm  (pu)>"
  Bus Creator/1 -> sm/1
  to W/1 -> Bus Creator/1  "Electrical Power (W)"
  Bus Selector/3 -> Bus Creator/4, to W1/1  "<Output active power   Peo (pu)>"
  Bus Selector/1 -> to W/1, Bus Creator/2  "<Electrical power  Pe (pu)>"
  Bus Selector/4 -> Bus Creator/5, to W2/1  "<Output reactive power  Qeo (pu)>"
  m/1 -> Bus Selector/1

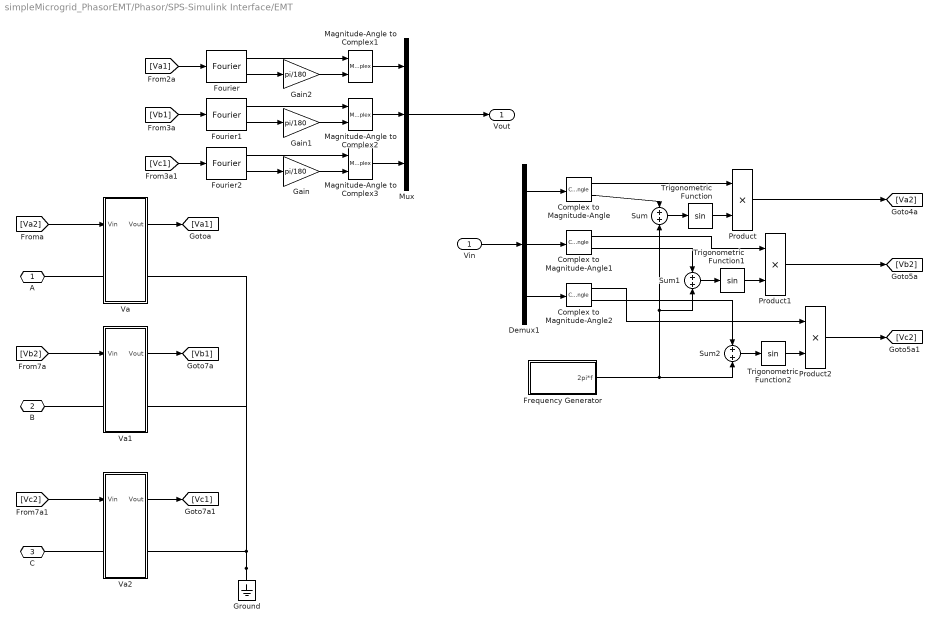
== system simpleMicrogrid_PhasorEMT/Phasor/SPS-Simulink Interface/EMT ==
  Vin : Inport
      settings: SignalType=complex
  Complex to Magnitude-Angle : ComplexToMagnitudeAngle
  Complex to Magnitude-Angle1 : ComplexToMagnitudeAngle
  Complex to Magnitude-Angle2 : ComplexToMagnitudeAngle
  Demux1 : Demux  Outputs=3
  Fourier : powerlib_meascontrol/Measurements/Fourier  Freq=60  n=1  InInit=[1, 0]  Ts=Ts
      settings: SourceProductName=Simscape Power Systems
  Fourier1 : powerlib_meascontrol/Measurements/Fourier  Freq=60  n=1  InInit=[1, 0]  Ts=Ts
      settings: SourceProductName=Simscape Power Systems
  Fourier2 : powerlib_meascontrol/Measurements/Fourier  Freq=60  n=1  InInit=[1, 0]  Ts=Ts
      settings: SourceProductName=Simscape Power Systems
  Frequency Generator : Subsystem  Variant=on  OverrideUsingVariant=Continuous
  Gain : Gain  Gain=pi/180
  Gain1 : Gain  Gain=pi/180
  Gain2 : Gain  Gain=pi/180
  Ground : powerlib/Elements/Ground  LConnTagsString=a
  Magnitude-Angle to Complex1 : MagnitudeAngleToComplex
  Magnitude-Angle to Complex2 : MagnitudeAngleToComplex
  Magnitude-Angle to Complex3 : MagnitudeAngleToComplex
  Mux : Mux  Inputs=3
  Product : Product
  Product1 : Product
  Product2 : Product
  Sum : Sum
  Sum1 : Sum
  Sum2 : Sum
  Trigonometric Function : Trigonometry
  Trigonometric Function1 : Trigonometry
  Trigonometric Function2 : Trigonometry
  Va : Subsystem
  Va1 : Subsystem
  Va2 : Subsystem
  A : PMIOPort  Port=1  Side=Right
  B : PMIOPort  Port=2  Side=Right
  C : PMIOPort  Port=3  Side=Right
  Vout : Outport
      settings: SignalType=complex
  wires:
  Complex to Magnitude-Angle2/2 -> Sum2/1
  Sum2/1 -> Trigonometric Function2/1
  Trigonometric Function2/1 -> Product2/2
  Complex to Magnitude-Angle2/1 -> Product2/1
  Complex to Magnitude-Angle1/1 -> Product1/1
  Trigonometric Function1/1 -> Product1/2
  Sum1/1 -> Trigonometric Function1/1
  Complex to Magnitude-Angle1/2 -> Sum1/1
  Frequency Generator/1(2pi*f) -> Sum/2, Sum1/2, Sum2/2
  Complex to Magnitude-Angle/2 -> Sum/1
  Sum/1 -> Trigonometric Function/1
  Trigonometric Function/1 -> Product/2
  Complex to Magnitude-Angle/1 -> Product/1
  Demux1/3 -> Complex to Magnitude-Angle2/1
  Demux1/2 -> Complex to Magnitude-Angle1/1
  Demux1/1 -> Complex to Magnitude-Angle/1
  Gain2/1 -> Magnitude-Angle to Complex1/2
  Gain1/1 -> Magnitude-Angle to Complex2/2
  Gain/1 -> Magnitude-Angle to Complex3/2
  Magnitude-Angle to Complex2/1 -> Mux/2
  Magnitude-Angle to Complex3/1 -> Mux/3
  Fourier2/2 -> Gain/1
  Fourier2/1 -> Magnitude-Angle to Complex3/1
  Fourier1/2 -> Gain1/1
  Fourier1/1 -> Magnitude-Angle to Complex2/1
  Magnitude-Angle to Complex1/1 -> Mux/1
  Fourier/1 -> Magnitude-Angle to Complex1/1
  Fourier/2 -> Gain2/1
  [Vc1] -> Fourier2/1
  [Vb1] -> Fourier1/1
  [Va1] -> Fourier/1
  Vin/1 -> Demux1/1
  Mux/1 -> Vout/1
  Product/1 -> [Va2]
  Product1/1 -> [Vb2]
  [Va2] -> Va/1(Vin)
  Va/1(Vout) -> [Va1]
  [Vb2] -> Va1/1(Vin)
  Va1/1(Vout) -> [Vb1]
  Va2/1(Vout) -> [Vc1]
  [Vc2] -> Va2/1(Vin)
  Product2/1 -> [Vc2]
  connections:
  Ground/LConn1 -- Va2/RConn1 -- Va1/RConn1 -- Va/RConn1
  Va/LConn1 -- A/RConn1
  Va1/LConn1 -- B/RConn1
  Va2/LConn1 -- C/RConn1

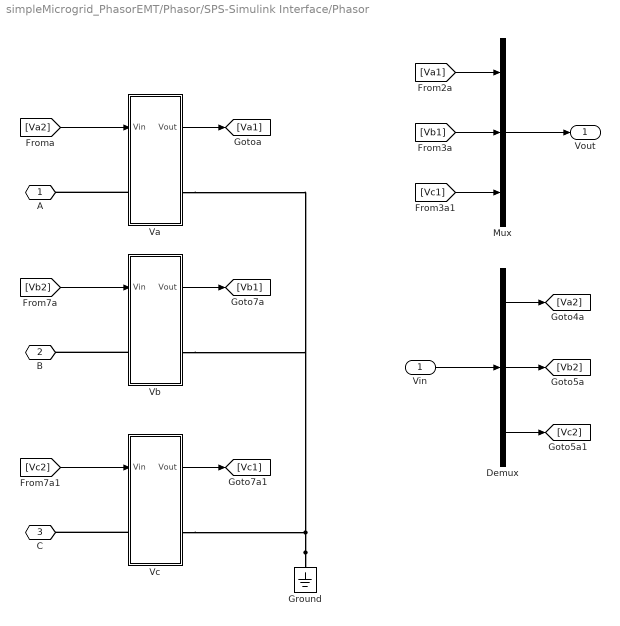
== system simpleMicrogrid_PhasorEMT/Phasor/SPS-Simulink Interface/Phasor ==
  Vin : Inport
  Demux : Demux  Outputs=3
  Ground : powerlib/Elements/Ground  LConnTagsString=a
  Mux : Mux  Inputs=3
  Va : Subsystem
  Vb : Subsystem
  Vc : Subsystem
  A : PMIOPort  Port=1  Side=Right
  B : PMIOPort  Port=2  Side=Right
  C : PMIOPort  Port=3  Side=Right
  Vout : Outport
  wires:
  Vin/1 -> Demux/1
  Mux/1 -> Vout/1
  [Va1] -> Mux/1
  [Vb1] -> Mux/2
  Demux/1 -> [Va2]
  Demux/2 -> [Vb2]
  [Va2] -> Va/1(Vin)
  Va/1(Vout) -> [Va1]
  [Vb2] -> Vb/1(Vin)
  Vb/1(Vout) -> [Vb1]
  Vc/1(Vout) -> [Vc1]
  [Vc2] -> Vc/1(Vin)
  [Vc1] -> Mux/3
  Demux/3 -> [Vc2]
  connections:
  Ground/LConn1 -- Vc/RConn1 -- Vb/RConn1 -- Va/RConn1
  Va/LConn1 -- A/RConn1
  Vb/LConn1 -- B/RConn1
  Vc/LConn1 -- C/RConn1

== system simpleMicrogrid_PhasorEMT/Phasor/Variable Load/Dynamic Load Control ==
  P0 : Inport
  Fcn : Fcn  Expr=sqrt(1/u(1)-1)
  Mux : Mux  Inputs=2
  Product : Product
  Summer1 : Constant  Value=PF
  PQ : Outport
  wires:
  Summer1/1 -> Fcn/1
  Fcn/1 -> Product/2
  P0/1 -> Product/1, Mux/1
  Mux/1 -> PQ/1
  Product/1 -> Mux/2  "Qo"

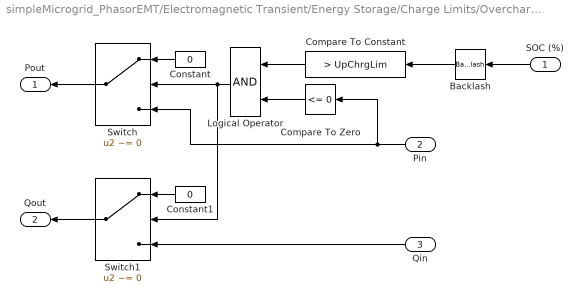
== system simpleMicrogrid_PhasorEMT/Electromagnetic Transient/Energy Storage/Charge Limits/Overcharge Check ==
  SOC (%) : Inport
  Pin : Inport  Port=2
  Qin : Inport  Port=3
  Backlash : Backlash  BacklashWidth=1e-3  InitialOutput=Initial_kWh_pc  ZeroCross=off
  Compare To Constant : simulink/Logic and Bit Operations/Compare To Constant  relop=>  const=UpChrgLim  OutDataTypeStr=boolean
  Compare To Zero : simulink/Logic and Bit Operations/Compare To Zero  relop=<=  OutDataTypeStr=boolean
  Constant : Constant  Value=0
  Constant1 : Constant  Value=0
  Logical Operator : Logic  AllPortsSameDT=off  OutDataTypeStr=boolean
  Switch : Switch  Criteria=u2 ~= 0
  Switch1 : Switch  Criteria=u2 ~= 0
  Pout : Outport
  Qout : Outport  Port=2
  wires:
  Backlash/1 -> Compare To Constant/1
  Switch1/1 -> Qout/1
  Constant1/1 -> Switch1/1
  Qin/1 -> Switch1/3
  Compare To Zero/1 -> Logical Operator/2
  Switch/1 -> Pout/1
  Pin/1 -> Switch/3, Compare To Zero/1
  SOC (%)/1 -> Backlash/1
  Constant/1 -> Switch/1
  Logical Operator/1 -> Switch/2, Switch1/2
  Compare To Constant/1 -> Logical Operator/1

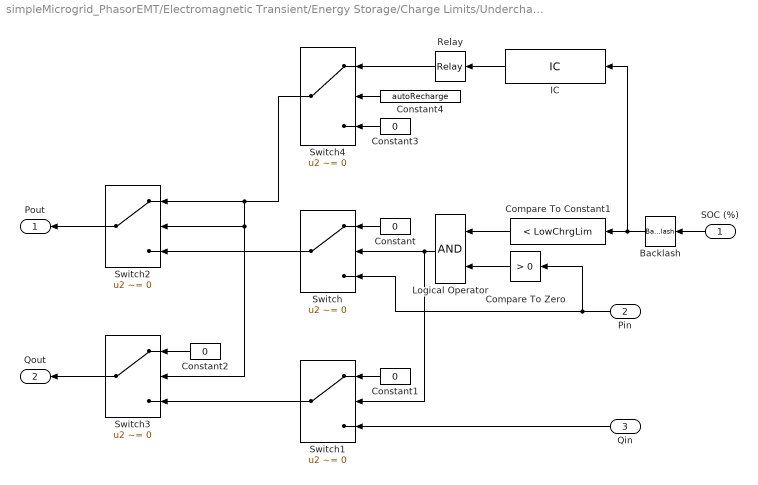
== system simpleMicrogrid_PhasorEMT/Electromagnetic Transient/Energy Storage/Charge Limits/Undercharge Check ==
  SOC (%) : Inport
  Pin : Inport  Port=2
  Qin : Inport  Port=3
  Backlash : Backlash  BacklashWidth=1e-3  InitialOutput=Initial_kWh_pc  ZeroCross=off
  Compare To Constant1 : simulink/Logic and Bit Operations/Compare To Constant  relop=<  const=LowChrgLim  OutDataTypeStr=boolean
  Compare To Zero : simulink/Logic and Bit Operations/Compare To Zero  relop=>  OutDataTypeStr=boolean
  Constant{,1..3} (4 alike) : Constant  Value=0
  Constant4 : Constant  Value=autoRecharge
  IC : InitialCondition  Value=RechargeSOC
  Logical Operator : Logic  AllPortsSameDT=off  OutDataTypeStr=boolean
  Relay : Relay  OnSwitchValue=RechargeSOC  OffSwitchValue=LowChrgLim  OnOutputValue=0  OffOutputValue=-Precharge/100*Pnom
  Switch{,1..4} (5 alike) : Switch  Criteria=u2 ~= 0
  Pout : Outport
  Qout : Outport  Port=2
  wires:
  Constant4/1 -> Switch4/2
  Constant3/1 -> Switch4/3
  Relay/1 -> Switch4/1
  Constant2/1 -> Switch3/1
  Switch1/1 -> Switch3/3
  Switch3/1 -> Qout/1
  Switch2/1 -> Pout/1
  Switch/1 -> Switch2/3
  IC/1 -> Relay/1
  Switch4/1 -> Switch3/2, Switch2/2, Switch2/1
  Backlash/1 -> Compare To Constant1/1, IC/1
  Qin/1 -> Switch1/3
  Constant1/1 -> Switch1/1
  Compare To Constant1/1 -> Logical Operator/1
  Logical Operator/1 -> Switch1/2, Switch/2
  Constant/1 -> Switch/1
  SOC (%)/1 -> Backlash/1
  Pin/1 -> Compare To Zero/1, Switch/3
  Compare To Zero/1 -> Logical Operator/2

== system simpleMicrogrid_PhasorEMT/Electromagnetic Transient/Energy Storage/Stored Energy Calculation (%)/Filter ==
  In1 : Inport
  1/T6 : Gain  Gain=1/Tf
  Discrete-Time Integrator : DiscreteIntegrator  SampleTime=Ts  ICPrevOutput=DiscIntNeverNeededParam  ICPrevScaledInput=DiscIntNeverNeededParam
  Sum1 : Sum  Inputs=|+-
  Out1 : Outport
  wires:
  Sum1/1 -> 1/T6/1
  Discrete-Time Integrator/1 -> Sum1/2, Out1/1
  In1/1 -> Sum1/1
  1/T6/1 -> Discrete-Time Integrator/1

== system simpleMicrogrid_PhasorEMT/Electromagnetic Transient/SPS-Simulink Interface/EMT/Frequency Generator ==
  Continuous : Subsystem  VariantControl=Continuous
  Discrete : Subsystem  VariantControl=Discrete
  2pi*f : Outport

== system simpleMicrogrid_PhasorEMT/Electromagnetic Transient/SPS-Simulink Interface/EMT/Va ==
  Vin : Inport
  Controlled Voltage Source : powerlib/Electrical Sources/Controlled Voltage Source  Initialize=off  Source_Type=AC  Amplitude=0  Phase=0  Frequency=0  Measurements=None
  Gain : Gain  Gain=kv
  Series RLC Branch : powerlib/Elements/Series RLC Branch  LConnTagsString=__new0  RConnTagsString=__new0  BranchType=R  Resistance=Rs  Inductance=Ls  SetiL0=off  InitialCurrent=0  Capacitance=Ls  Setx0=off  InitialVoltage=0  Measurements=None
  Sum : Sum
  Voltage Measurement : powerlib/Measurements/Voltage Measurement  PhasorSimulation=off  OutputType=Complex  PSBequivalent=0
  Voltage Measurement1 : powerlib/Measurements/Voltage Measurement  PhasorSimulation=off  OutputType=Complex  PSBequivalent=0
  + : PMIOPort  Port=1  Side=Left
  - : PMIOPort  Port=2  Side=Right
  Vout : Outport
  wires:
  Voltage Measurement/1 -> Sum/2
  Voltage Measurement1/1 -> Gain/1
  Vin/1 -> Controlled Voltage Source/1
  Sum/1 -> Vout/1
  Gain/1 -> Sum/1
  connections:
  Voltage Measurement/LConn2 -- -/RConn1 -- Controlled Voltage Source/LConn1
  Voltage Measurement1/LConn1 -- Voltage Measurement/LConn1 -- Series RLC Branch/LConn1 -- +/RConn1
  Controlled Voltage Source/RConn1 -- Voltage Measurement1/LConn2 -- Series RLC Branch/RConn1

== system simpleMicrogrid_PhasorEMT/Electromagnetic Transient/SPS-Simulink Interface/EMT/Va1 ==
  Vin : Inport
  Controlled Voltage Source : powerlib/Electrical Sources/Controlled Voltage Source  Initialize=off  Source_Type=AC  Amplitude=0  Phase=0  Frequency=0  Measurements=None
  Gain : Gain  Gain=kv
  Series RLC Branch : powerlib/Elements/Series RLC Branch  LConnTagsString=__new0  RConnTagsString=__new0  BranchType=R  Resistance=Rs  Inductance=Ls  SetiL0=off  InitialCurrent=0  Capacitance=Ls  Setx0=off  InitialVoltage=0  Measurements=None
  Sum : Sum
  Voltage Measurement : powerlib/Measurements/Voltage Measurement  PhasorSimulation=off  OutputType=Complex  PSBequivalent=0
  Voltage Measurement1 : powerlib/Measurements/Voltage Measurement  PhasorSimulation=off  OutputType=Complex  PSBequivalent=0
  + : PMIOPort  Port=1  Side=Left
  - : PMIOPort  Port=2  Side=Right
  Vout : Outport
  wires:
  Gain/1 -> Sum/1
  Sum/1 -> Vout/1
  Vin/1 -> Controlled Voltage Source/1
  Voltage Measurement1/1 -> Gain/1
  Voltage Measurement/1 -> Sum/2
  connections:
  Series RLC Branch/RConn1 -- Voltage Measurement1/LConn2 -- Controlled Voltage Source/RConn1
  +/RConn1 -- Series RLC Branch/LConn1 -- Voltage Measurement/LConn1 -- Voltage Measurement1/LConn1
  Controlled Voltage Source/LConn1 -- -/RConn1 -- Voltage Measurement/LConn2

== system simpleMicrogrid_PhasorEMT/Electromagnetic Transient/SPS-Simulink Interface/EMT/Va2 ==
  Vin : Inport
  Controlled Voltage Source : powerlib/Electrical Sources/Controlled Voltage Source  Initialize=off  Source_Type=AC  Amplitude=0  Phase=0  Frequency=0  Measurements=None
  Gain : Gain  Gain=kv
  Series RLC Branch : powerlib/Elements/Series RLC Branch  LConnTagsString=__new0  RConnTagsString=__new0  BranchType=R  Resistance=Rs  Inductance=Ls  SetiL0=off  InitialCurrent=0  Capacitance=Ls  Setx0=off  InitialVoltage=0  Measurements=None
  Sum : Sum
  Voltage Measurement : powerlib/Measurements/Voltage Measurement  PhasorSimulation=off  OutputType=Complex  PSBequivalent=0
  Voltage Measurement1 : powerlib/Measurements/Voltage Measurement  PhasorSimulation=off  OutputType=Complex  PSBequivalent=0
  + : PMIOPort  Port=1  Side=Left
  - : PMIOPort  Port=2  Side=Right
  Vout : Outport
  wires:
  Voltage Measurement/1 -> Sum/2
  Voltage Measurement1/1 -> Gain/1
  Vin/1 -> Controlled Voltage Source/1
  Sum/1 -> Vout/1
  Gain/1 -> Sum/1
  connections:
  Voltage Measurement/LConn2 -- -/RConn1 -- Controlled Voltage Source/LConn1
  Voltage Measurement1/LConn1 -- Voltage Measurement/LConn1 -- Series RLC Branch/LConn1 -- +/RConn1
  Controlled Voltage Source/RConn1 -- Voltage Measurement1/LConn2 -- Series RLC Branch/RConn1

== system simpleMicrogrid_PhasorEMT/Electromagnetic Transient/SPS-Simulink Interface/Phasor/Va ==
  Vin : Inport
  Controlled Voltage Source : powerlib/Electrical Sources/Controlled Voltage Source  Initialize=off  Source_Type=AC  Amplitude=0  Phase=0  Frequency=0  Measurements=None
  Gain : Gain  Gain=kv
  Series RLC Branch : powerlib/Elements/Series RLC Branch  LConnTagsString=__new0  RConnTagsString=__new0  BranchType=R  Resistance=Rs  Inductance=1e-3  SetiL0=off  InitialCurrent=0  Capacitance=1e-6  Setx0=off  InitialVoltage=0  Measurements=None
  Sum : Sum
  Voltage Measurement : powerlib/Measurements/Voltage Measurement  PhasorSimulation=off  OutputType=Complex  PSBequivalent=0
  Voltage Measurement1 : powerlib/Measurements/Voltage Measurement  PhasorSimulation=off  OutputType=Complex  PSBequivalent=0
  + : PMIOPort  Port=1  Side=Left
  - : PMIOPort  Port=2  Side=Right
  Vout : Outport
  wires:
  Gain/1 -> Sum/1
  Voltage Measurement/1 -> Sum/2
  Voltage Measurement1/1 -> Gain/1
  Vin/1 -> Controlled Voltage Source/1
  Sum/1 -> Vout/1
  connections:
  Voltage Measurement/LConn2 -- -/RConn1 -- Controlled Voltage Source/LConn1
  Voltage Measurement1/LConn1 -- Voltage Measurement/LConn1 -- Series RLC Branch/LConn1 -- +/RConn1
  Controlled Voltage Source/RConn1 -- Voltage Measurement1/LConn2 -- Series RLC Branch/RConn1

== system simpleMicrogrid_PhasorEMT/Electromagnetic Transient/SPS-Simulink Interface/Phasor/Vb ==
  Vin : Inport
  Controlled Voltage Source : powerlib/Electrical Sources/Controlled Voltage Source  Initialize=off  Source_Type=AC  Amplitude=0  Phase=0  Frequency=0  Measurements=None
  Gain : Gain  Gain=kv
  Series RLC Branch : powerlib/Elements/Series RLC Branch  LConnTagsString=__new0  RConnTagsString=__new0  BranchType=R  Resistance=Rs  Inductance=1e-3  SetiL0=off  InitialCurrent=0  Capacitance=1e-6  Setx0=off  InitialVoltage=0  Measurements=None
  Sum : Sum
  Voltage Measurement : powerlib/Measurements/Voltage Measurement  PhasorSimulation=off  OutputType=Complex  PSBequivalent=0
  Voltage Measurement1 : powerlib/Measurements/Voltage Measurement  PhasorSimulation=off  OutputType=Complex  PSBequivalent=0
  + : PMIOPort  Port=1  Side=Left
  - : PMIOPort  Port=2  Side=Right
  Vout : Outport
  wires:
  Sum/1 -> Vout/1
  Vin/1 -> Controlled Voltage Source/1
  Voltage Measurement1/1 -> Gain/1
  Voltage Measurement/1 -> Sum/2
  Gain/1 -> Sum/1
  connections:
  Series RLC Branch/RConn1 -- Voltage Measurement1/LConn2 -- Controlled Voltage Source/RConn1
  +/RConn1 -- Series RLC Branch/LConn1 -- Voltage Measurement/LConn1 -- Voltage Measurement1/LConn1
  Controlled Voltage Source/LConn1 -- -/RConn1 -- Voltage Measurement/LConn2
